simulink model "Read_lidar"  (R2020a)
settings: Solver=FixedStepAuto  StartTime=0.0  StopTime=inf  RelTol=1e-3
model workspace (MAT data in the model file):
  SL_ROS_VariableLengthArrays_MaxSizes.CommonInfo.ArrayTruncateAction = 'EmitWarning'
  SL_ROS_VariableLengthArrays_MaxSizes.MsgTypeMap = containers.Map
  SL_ROS_VariableLengthArrays_MaxSizes.MsgTypeMap.serialization.keys = {'sensor_msgs/CompressedImage', 'sensor_msgs/LaserScan'}
  SL_ROS_VariableLengthArrays_MaxSizes.MsgTypeMap.serialization.values{1}(1).PropertyName = 'Data'
  SL_ROS_VariableLengthArrays_MaxSizes.MsgTypeMap.serialization.values{1}(1).DataType = 'uint8'
  SL_ROS_VariableLengthArrays_MaxSizes.MsgTypeMap.serialization.values{1}(1).MaxLength = 200000
  SL_ROS_VariableLengthArrays_MaxSizes.MsgTypeMap.serialization.values{1}(2).PropertyName = 'Format'
  SL_ROS_VariableLengthArrays_MaxSizes.MsgTypeMap.serialization.values{1}(2).DataType = 'uint8'
  SL_ROS_VariableLengthArrays_MaxSizes.MsgTypeMap.serialization.values{1}(2).MaxLength = 128
  SL_ROS_VariableLengthArrays_MaxSizes.MsgTypeMap.serialization.values{2}(1).PropertyName = 'Intensities'
  SL_ROS_VariableLengthArrays_MaxSizes.MsgTypeMap.serialization.values{2}(1).DataType = 'single'
  SL_ROS_VariableLengthArrays_MaxSizes.MsgTypeMap.serialization.values{2}(1).MaxLength = 360
  SL_ROS_VariableLengthArrays_MaxSizes.MsgTypeMap.serialization.values{2}(2).PropertyName = 'Ranges'
  SL_ROS_VariableLengthArrays_MaxSizes.MsgTypeMap.serialization.values{2}(2).DataType = 'single'
  SL_ROS_VariableLengthArrays_MaxSizes.MsgTypeMap.serialization.values{2}(2).MaxLength = 360
  SL_ROS_VariableLengthArrays_MaxSizes.MsgTypeMap.serialization.uniformity = 0
  SL_ROS_VariableLengthArrays_MaxSizes.MsgTypeMap.serialization.keyType = 'char'
  SL_ROS_VariableLengthArrays_MaxSizes.MsgTypeMap.serialization.valueType = 'any'
undefined symbols (not defined in the file or in its folder): Angular, Linear
libraries: simulink_extras x4, robotlib x3, realtime_pacer_lib x2, vrlib x1, visiongeotforms x1, visionsinks x1
settings Model: Creator=20195009  LastModifiedBy=TruckLabPC2
settings OptimizationCC: EnhancedBackFolding=on  PassReuseOutputArgsAs=Individual arguments  ZeroExternalMemoryAtStartup=off  ZeroInternalMemoryAtStartup=off  MaxStackSize=64  OptimizeBlockOrder=speed  DifferentSizesBufferReuse=on  OptimizationCustomize=off  EfficientTunableParamExpr=on
settings DebuggingCC: ParameterTunabilityLossMsg=error  SFMachineParentedDataDiag=error
settings HardwareCC: ProdBitPerPointer=32  ProdBitPerSizeT=32  ProdBitPerPtrDiffT=32  ProdLargestAtomicFloat=None  ProdIntDivRoundTo=Undefined  ProdEndianess=Unspecified  ProdWordSize=32  ProdHWDeviceType=Generic->Unspecified (assume 32-bit Generic)
settings SFSimCC: MATLABDynamicMemAlloc=off
settings RTWCC: SystemTargetFile=ert.tlc  HardwareBoard=Robot Operating System (ROS)  TemplateMakefile=ert_default_tmf  Toolchain=Catkin  TargetLang=C++
settings CodeAppCC: ForceParamTrailComments=on  IgnoreCustomStorageClasses=off  OperatorAnnotations=on  SimulinkDataObjDesc=on  SFDataObjDesc=on  InsertBlockDesc=on

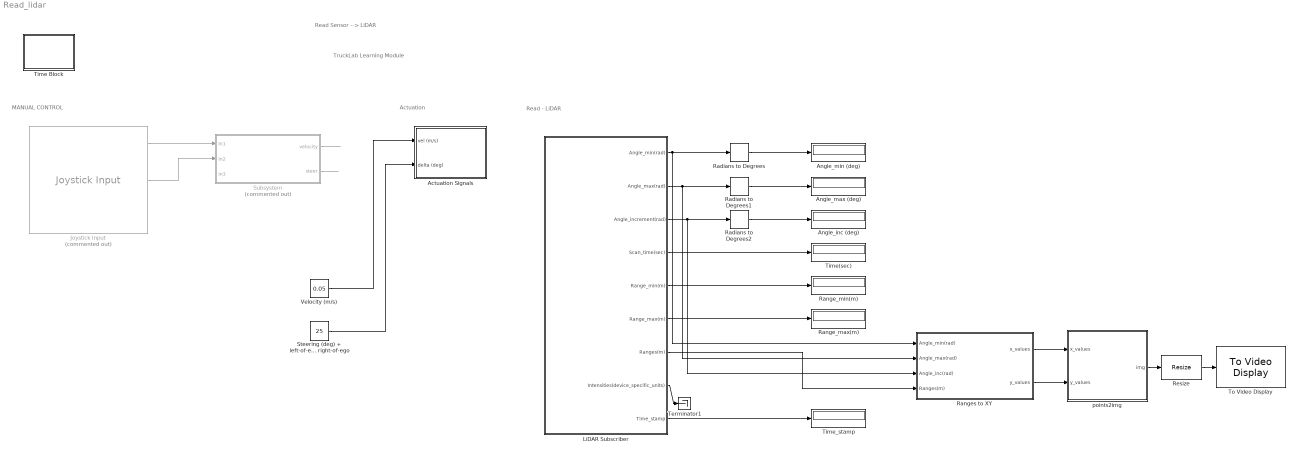
== system Read_lidar ==
  note: Read - LiDAR
  note: MANUAL CONTROL
  note: TruckLab Learning Module
  note: Actuation
  note: Read Sensor --> LiDAR
  Actuation Signals : Subsystem
  Angle_inc (deg) : Display
  Angle_max (deg) : Display
  Angle_min (deg) : Display
  Joystick Input : vrlib/Joystick Input  Commented=on  joyid=1  adjustports=on  forcefeed=off
  LiDAR Subscriber : Subsystem
  Radians to Degrees : simulink_extras/Transformations/Radians to Degrees
  Radians to Degrees1 : simulink_extras/Transformations/Radians to Degrees
  Radians to Degrees2 : simulink_extras/Transformations/Radians to Degrees
  Range_max(m) : Display
  Range_min(m) : Display
  Ranges to XY : Subsystem
  Resize : visiongeotforms/Resize  specify=Output size as a percentage of input size  rfactor=[100 100]  outCols=25  outRows=25  outRowsCols=[25 35]  interp_method=Bilinear  antialias=on  useROI=off  roiFlag=off  roundingMode=Nearest  overflowMode=on  prodOutputMode=Binary point scaling  prodOutputWordLength=32  prodOutputFracLength=10
      settings: SourceProductBaseCode=VP
  Steering (deg) + left-of-ego - right-of-ego : Constant  Value=25
  Subsystem : Subsystem  Commented=on
  Terminator1 : Terminator
  Time Block : Subsystem
  Time(sec) : Display
  Time_stamp : Display
  To Video Display : visionsinks/To Video Display  windowSizeMode=True size (1:1)  openAtMdlStart=on  fullScreen=off  videoWindowX=817  videoWindowY=234  saveWindowSize=off  videoWindowWidth=800  videoWindowHeight=800  inputColorFormat=RGB  inputType=Obsolete  imagePorts=One multidimensional signal  OutputDevice=On-screen video monitor  dataOrg=Column-major  isWindowOpen=off
  Velocity (m/s) : Constant  Value=0.05
  points2img : MATLAB Function  TreatAsAtomicUnit=on
  wires:
  LiDAR Subscriber/1(Angle_min(rad)) -> Ranges to XY/1(Angle_min(rad)), Radians to Degrees/1
  Radians to Degrees/1 -> Angle_min (deg)/1
  LiDAR Subscriber/2(Angle_max(rad)) -> Radians to Degrees1/1, Ranges to XY/2(Angle_max(rad))
  Radians to Degrees1/1 -> Angle_max (deg)/1
  LiDAR Subscriber/3(Angle_increment(rad)) -> Radians to Degrees2/1, Ranges to XY/3(Angle_inc(rad))
  Radians to Degrees2/1 -> Angle_inc (deg)/1
  LiDAR Subscriber/4(Scan_time(sec)) -> Time(sec)/1
  LiDAR Subscriber/5(Range_min(m)) -> Range_min(m)/1
  LiDAR Subscriber/6(Range_max(m)) -> Range_max(m)/1
  LiDAR Subscriber/7(Ranges(m)) -> Ranges to XY/4(Ranges(m))
  LiDAR Subscriber/9(Time_stamp) -> Time_stamp/1
  LiDAR Subscriber/8(Intensities(device_specific_units)) -> Terminator1/1
  Ranges to XY/2(y_values) -> points2img/2(y_values)
  Ranges to XY/1(x_values) -> points2img/1(x_values)
  points2img/1(img) -> Resize/1
  Resize/1 -> To Video Display/1
  Subsystem/1(velocity) -> ?
  Velocity (m/s)/1 -> Actuation Signals/1(vel (m/s))
  ? -> Subsystem/3(In3)
  Subsystem/2(steer) -> ?
  Joystick Input/1 -> Subsystem/1(In1)
  Steering (deg) + left-of-ego - right-of-ego/1 -> Actuation Signals/2(delta (deg))
  Joystick Input/2 -> Subsystem/2(In2)

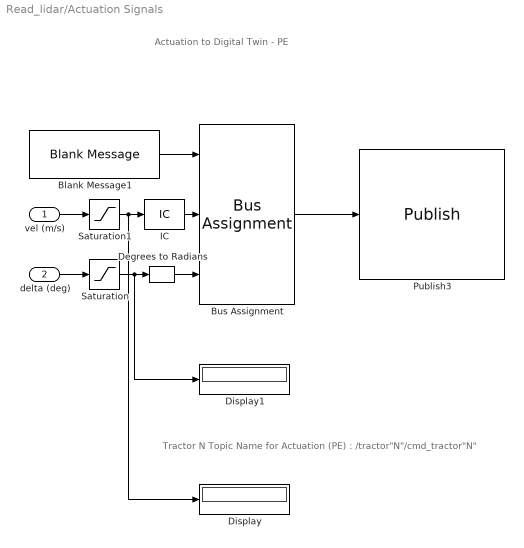
== system Read_lidar/Actuation Signals ==
  note: Tractor N Topic Name for Actuation (PE) : /tractor"N"/cmd_tractor"N"
  note: Actuation to Digital Twin - PE
  vel (m/s) : Inport
  delta (deg) : Inport  Port=2
  Blank Message1 : robotlib/Blank Message  messageClass=Message  entityType=geometry_msgs/Twist  messageType=geometry_msgs/Twist  SampleTime=0.01
  Bus Assignment : BusAssignment  DialogController=Simulink.DDGSource_BusAssignment  AssignedSignals=Linear.X,Angular.Z
  Degrees to Radians : simulink_extras/Transformations/Degrees to Radians
  Display : Display
  Display1 : Display
  IC : InitialCondition  Value=0
  Publish3 : robotlib/Publish  topicSource=Select from ROS network  topic=/tractor1/cmd_tractor1  messageType=geometry_msgs/Twist  messageQueueLength=1
      link override SinkBlock: ROSTopic=/cmd_vel  ROSMessageType=geometry_msgs/Twist  SLBusName=SL_Bus_TruckLab_MannualDrivingROS1_geometry_msgs_Twist  ModelName=TruckLab_MannualDrivingROS1  BlockId=Pub_TruckLab_MannualDrivingROS1_402
  Saturation : Saturate  UpperLimit=25  LowerLimit=-25
  Saturation1 : Saturate  UpperLimit=0.28  LowerLimit=-0.28
  wires:
  vel (m/s)/1 -> Saturation1/1
  IC/1 -> Bus Assignment/2
  Bus Assignment/1 -> Publish3/1
  Degrees to Radians/1 -> Bus Assignment/3
  Blank Message1/1 -> Bus Assignment/1
  delta (deg)/1 -> Saturation/1
  Saturation/1 -> Display1/1, Degrees to Radians/1
  Saturation1/1 -> Display/1, IC/1

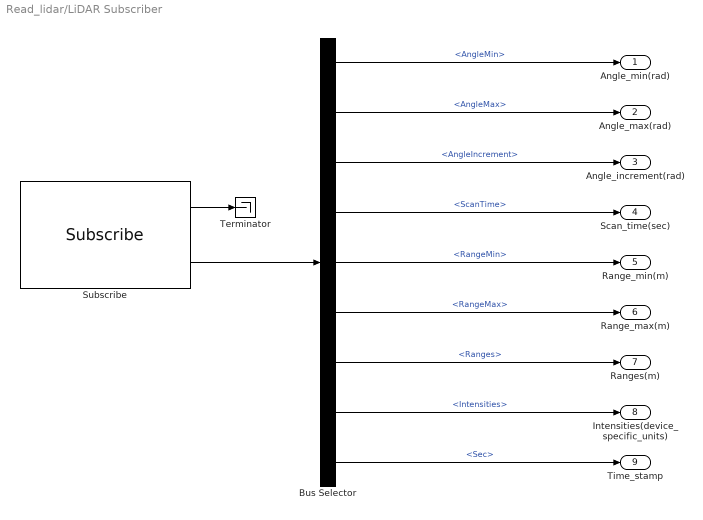
== system Read_lidar/LiDAR Subscriber ==
  Bus Selector : BusSelector  OutputSignals=AngleMin,AngleMax,AngleIncrement,ScanTime,RangeMin,RangeMax,Ranges,Intensities,Header.Stamp.Sec
  Subscribe : robotlib/Subscribe  topicSource=Select from ROS network  topic=/DC_1/TRACTOR_1/LIDAR_1/lidarscanfull  messageType=sensor_msgs/LaserScan  sampleTime=-1  messageQueueLength=1
  Terminator : Terminator
  Angle_min(rad) : Outport
  Angle_max(rad) : Outport  Port=2
  Angle_increment(rad) : Outport  Port=3
  Scan_time(sec) : Outport  Port=4
  Range_min(m) : Outport  Port=5
  Range_max(m) : Outport  Port=6
  Ranges(m) : Outport  Port=7
  Intensities(device_specific_units) : Outport  Port=8
  Time_stamp : Outport  Port=9
  wires:
  Subscribe/1 -> Terminator/1
  Subscribe/2 -> Bus Selector/1
  Bus Selector/1 -> Angle_min(rad)/1  "<AngleMin>"
  Bus Selector/2 -> Angle_max(rad)/1  "<AngleMax>"
  Bus Selector/5 -> Range_min(m)/1  "<RangeMin>"
  Bus Selector/6 -> Range_max(m)/1  "<RangeMax>"
  Bus Selector/8 -> Intensities(device_specific_units)/1  "<Intensities>"
  Bus Selector/9 -> Time_stamp/1  "<Sec>"
  Bus Selector/3 -> Angle_increment(rad)/1  "<AngleIncrement>"
  Bus Selector/7 -> Ranges(m)/1  "<Ranges>"
  Bus Selector/4 -> Scan_time(sec)/1  "<ScanTime>"

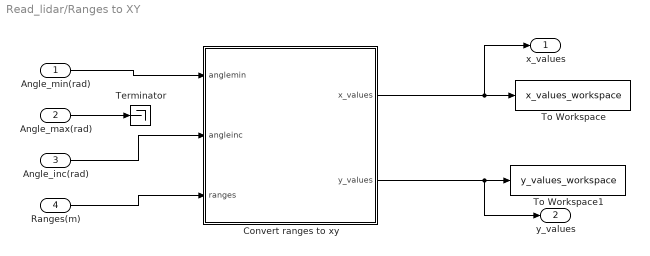
== system Read_lidar/Ranges to XY ==
  Angle_min(rad) : Inport
  Angle_max(rad) : Inport  Port=2
  Angle_inc(rad) : Inport  Port=3
  Ranges(m) : Inport  Port=4
  Convert ranges to xy : MATLAB Function  TreatAsAtomicUnit=on
  Terminator : Terminator
  To Workspace : ToWorkspace  VariableName=x_values_workspace  SampleTime=-1
  To Workspace1 : ToWorkspace  VariableName=y_values_workspace  SampleTime=-1
  x_values : Outport
  y_values : Outport  Port=2
  wires:
  Angle_min(rad)/1 -> Convert ranges to xy/1(anglemin)
  Angle_max(rad)/1 -> Terminator/1
  Angle_inc(rad)/1 -> Convert ranges to xy/2(angleinc)
  Ranges(m)/1 -> Convert ranges to xy/3(ranges)
  Convert ranges to xy/1(x_values) -> x_values/1, To Workspace/1
  Convert ranges to xy/2(y_values) -> y_values/1, To Workspace1/1

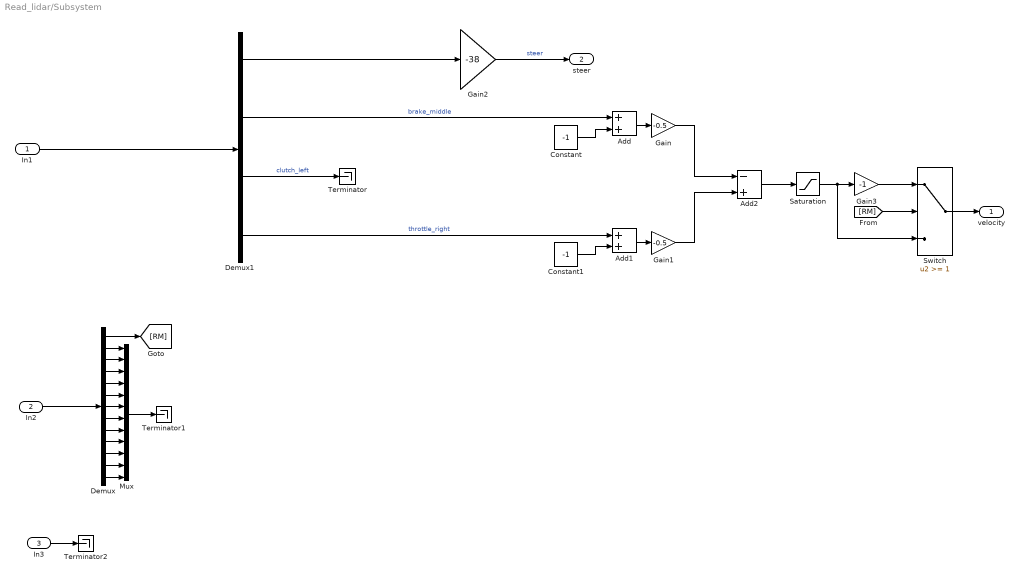
== system Read_lidar/Subsystem ==
  In1 : Inport
  In2 : Inport  Port=2
  In3 : Inport  Port=3
  Add : Sum
  Add1 : Sum
  Add2 : Sum  Inputs=-+
  Constant : Constant  Value=-1
  Constant1 : Constant  Value=-1
  Demux : Demux  Outputs=13
  Demux1 : Demux
  Gain : Gain  Gain=-0.5
  Gain1 : Gain  Gain=-0.5
  Gain2 : Gain  Gain=-38
  Gain3 : Gain  Gain=-1
  Mux : Mux  Inputs=12
  Saturation : Saturate  UpperLimit=5  LowerLimit=0
  Switch : Switch  Threshold=1
  Terminator : Terminator
  Terminator1 : Terminator
  Terminator2 : Terminator
  velocity : Outport
  steer : Outport  Port=2
  wires:
  [RM] -> Switch/2
  Gain3/1 -> Switch/1
  Demux1/4 -> Add1/1  "throttle_right"
  Switch/1 -> velocity/1
  Demux/1 -> [RM]
  Demux1/3 -> Terminator/1  "clutch_left"
  Mux/1 -> Terminator1/1
  In1/1 -> Demux1/1
  In2/1 -> Demux/1
  Demux/6 -> Mux/5
  Demux1/1 -> Gain2/1
  Demux/8 -> Mux/7
  In3/1 -> Terminator2/1
  Constant1/1 -> Add1/2
  Constant/1 -> Add/2
  Demux/9 -> Mux/8
  Demux/12 -> Mux/11
  Demux/5 -> Mux/4
  Demux/3 -> Mux/2
  Demux/10 -> Mux/9
  Gain2/1 -> steer/1  "steer"
  Gain1/1 -> Add2/2
  Add/1 -> Gain/1
  Demux1/2 -> Add/1  "brake_middle"
  Add2/1 -> Saturation/1
  Demux/7 -> Mux/6
  Demux/11 -> Mux/10
  Saturation/1 -> Switch/3, Gain3/1
  Demux/2 -> Mux/1
  Add1/1 -> Gain1/1
  Gain/1 -> Add2/1
  Demux/13 -> Mux/12
  Demux/4 -> Mux/3

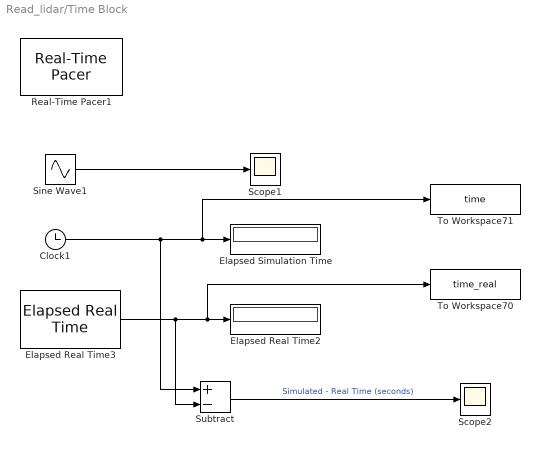
== system Read_lidar/Time Block ==
  Clock1 : Clock
  Elapsed Real Time2 : Display
      settings: Decimation=2
  Elapsed Real Time3 : realtime_pacer_lib/Elapsed Real Time
  Elapsed Simulation Time : Display
      settings: Decimation=2
  Real-Time Pacer1 : realtime_pacer_lib/Real-Time Pacer  simTimePerRealTime=1
  Scope1 : Scope
  Scope2 : Scope
  Sine Wave1 : Sin  Frequency=2*pi*0.5  SampleTime=0
  Subtract : Sum  Inputs=+-
  To Workspace70 : ToWorkspace  VariableName=time_real  SampleTime=-1
  To Workspace71 : ToWorkspace  VariableName=time  SampleTime=-1
  wires:
  Subtract/1 -> Scope2/1  "Simulated - Real Time (seconds)"
  Elapsed Real Time3/1 -> Elapsed Real Time2/1, To Workspace70/1, Subtract/2
  Sine Wave1/1 -> Scope1/1
  Clock1/1 -> Subtract/1, Elapsed Simulation Time/1, To Workspace71/1

== matlab function Read_lidar/Ranges to XY/Convert ranges to xy ==
  data: anglemin input; x_values output; angleinc input; ranges input; y_values output
function [x_values, y_values] = fcn(anglemin, angleinc, ranges)
angle_min = double(anglemin);
angle_inc = double(angleinc);
angles=double(zeros(numel(ranges),1));
for i=1:numel(ranges)
    angles(i) = double(angle_min) + double(i-1)*(angle_inc);
end

x_values = ranges.*cos(angles);
y_values = ranges.*sin(angles);

== matlab function Read_lidar/points2img ==
  data: img output; x_values input; y_values input
function img = fcn(x_values, y_values)
img = ones(800, 800)*255;
delta = 2;
delta_ego = 5;
% iterate over these points, and set up a primitive grid map
for i=1:numel(x_values)
    % (800, 800) pixels = (8m, 8m)
    m_to_px = 100;
    x = x_values(i);
    y = y_values(i);
    
    px_x = floor(x * m_to_px);
    px_y = floor(y * m_to_px);
    
    ind_min_x = max(1, px_x-delta+400);
    ind_max_x = min(800, px_x+delta+400);
    
    ind_min_y = max(1, px_y-delta+400);
    ind_max_y = min(800, px_y+delta+400);
    
    img(ind_min_x:ind_max_x, ind_min_y:ind_max_y) = 0;
    img(400-delta_ego:400+delta_ego, 400-delta_ego:400+delta_ego) = 0;
end
